simulink model "lti_id_0"  (R2018a)
settings: Solver=FixedStepAuto  StartTime=0.0  StopTime=5  FixedStep=0.0001  RelTol=1e-3
values from neighbouring files (symbols this model uses):
  b_eq = b_m + b_l/r^2    (= 1.5637748692e-05)    [PMSM_AyME.m]    (also in estabilidad_open_loop.m)
  J_eq = J_m + J_l/r^2    (= 5.65099476805e-06)    [PMSM_AyME.m]    (also in estabilidad_open_loop.m)
  L_q = 5.8E-3    (= 0.0058)    [PMSM_AyME.m]    (also in estabilidad_open_loop.m)
  lambda_m = 0.01546    [PMSM_AyME.m]    (also in estabilidad_open_loop.m)
  Pp = 3    [PMSM_AyME.m]    (also in estabilidad_open_loop.m)
  R_cq = -p_i*L_q    (= 29)    [PMSM_AyME.m]
  R_s = 1.02    [PMSM_AyME.m]    (also in estabilidad_open_loop.m)
settings Model: Creator=emiliano  LastModifiedBy=gino

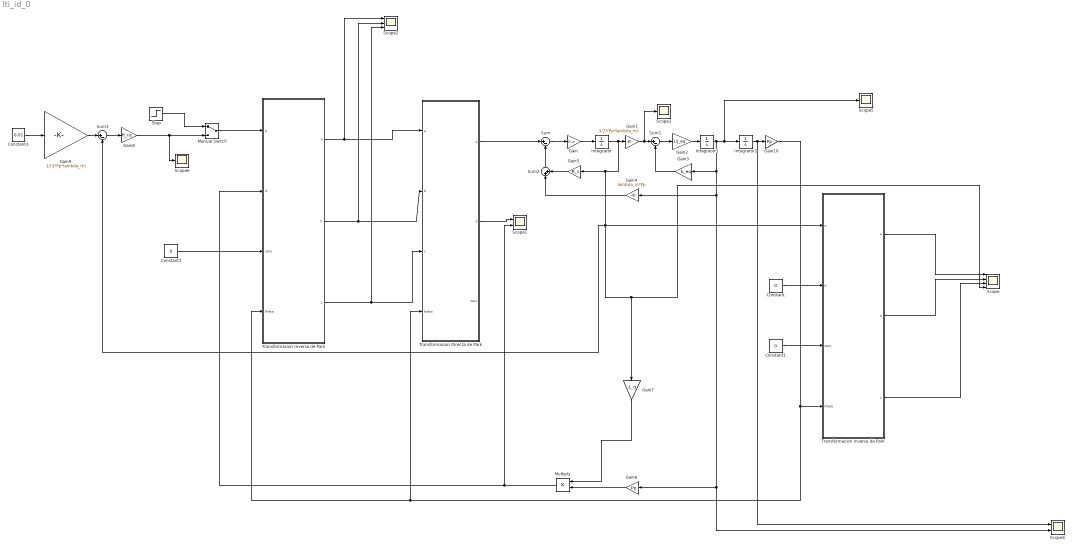
== system lti_id_0 ==
  Constant : Constant  Value=0
  Constant1 : Constant  Value=0
  Constant2 : Constant  Value=0
  Constant3 : Constant  Value=0.01
  Gain : Gain  Gain=1/L_q
  Gain1 : Gain  Gain=3/2*(Pp*lambda_m)
  Gain10 : Gain  Gain=Pp
  Gain2 : Gain  Gain=1/J_eq
  Gain3 : Gain  Gain=b_eq
  Gain4 : Gain  Gain=lambda_m*Pp
  Gain5 : Gain  Gain=R_s
  Gain6 : Gain  Gain=Pp
  Gain7 : Gain  Gain=-L_q
  Gain8 : Gain  Gain=R_cq
  Gain9 : Gain  Gain=2/(3*Pp*lambda_m)
  Integrator : Integrator
  Integrator1 : Integrator
  Integrator2 : Integrator
  Manual Switch : ManualSwitch
  Multiply : Product
  Scope : Scope  NumInputPorts=4
  Scope1 : Scope  NumInputPorts=2
  Scope2 : Scope  NumInputPorts=3
  Scope3 : Scope
  Scope4 : Scope  NumInputPorts=2
  Scope5 : Scope
  Scope6 : Scope
  Step : Step  After=20  SampleTime=0
  Sum : Sum  Inputs=|+-
  Sum1 : Sum  Inputs=|+-
  Sum2 : Sum  Inputs=|++
  Sum3 : Sum  Inputs=|+-
  Transformacion Directa de Park : MATLAB Function  TreatAsAtomicUnit=on
  Transformacion Inversa de Park : MATLAB Function  TreatAsAtomicUnit=on
  "Transformacion Inversa de Park " : MATLAB Function  TreatAsAtomicUnit=on
  wires:
  Sum/1 -> Gain/1
  Gain/1 -> Integrator/1
  Gain1/1 -> Scope3/1, Sum1/1
  Sum1/1 -> Gain2/1
  Gain2/1 -> Integrator1/1
  Integrator1/1 -> Scope4/2, Gain6/1, Gain4/1, Gain3/1, Scope5/1, Integrator2/1
  Gain3/1 -> Sum1/2
  Gain5/1 -> Sum2/2
  Sum2/1 -> Sum/2
  Gain4/1 -> Sum2/1
  Transformacion Directa de Park/1(q) -> Sum/1
  Integrator/1 -> Sum3/2, Scope/4, Gain7/1, Transformacion Inversa de Park/1(q), Gain5/1, Gain1/1
  Constant/1 -> Transformacion Inversa de Park/2(d)
  Constant1/1 -> Transformacion Inversa de Park/3(zero)
  Transformacion Inversa de Park/1(a) -> Scope/1
  Transformacion Inversa de Park/2(b) -> Scope/2
  Transformacion Inversa de Park/3(c) -> Scope/3
  Gain6/1 -> Multiply/2
  Gain7/1 -> Multiply/1
  Multiply/1 -> Scope1/2, "Transformacion Inversa de Park "/2(d)
  Constant2/1 -> "Transformacion Inversa de Park "/3(zero)
  Sum3/1 -> Gain8/1
  Constant3/1 -> Gain9/1
  Gain9/1 -> Sum3/1
  Transformacion Directa de Park/2(d) -> Scope1/1
  Gain10/1 -> Transformacion Directa de Park/4(theta), "Transformacion Inversa de Park "/4(theta), Transformacion Inversa de Park/4(theta)
  "Transformacion Inversa de Park "/1(a) -> Transformacion Directa de Park/1(a), Scope2/1
  "Transformacion Inversa de Park "/3(c) -> Transformacion Directa de Park/3(c), Scope2/3
  "Transformacion Inversa de Park "/2(b) -> Transformacion Directa de Park/2(b), Scope2/2
  Integrator2/1 -> Scope4/1, Gain10/1
  Manual Switch/1 -> "Transformacion Inversa de Park "/1(q)
  Gain8/1 -> Scope6/1, Manual Switch/2
  Step/1 -> Manual Switch/1

== matlab function lti_id_0/Transformacion Inversa de Park  ==
  data: q input; a output; d input; zero input; theta input; b output; c output
function [a, b, c] = inverse_park_transformation(q, d, zero, theta)
%Transformación inversa de Park
 
abc = [cos(theta)               sin(theta)              1
        cos(theta - 2*pi/3)     sin(theta - 2*pi/3)     1
        cos(theta + 2*pi/3)     sin(theta + 2*pi/3)     1] ...
    *   [q
        d
        zero];

a = abc(1);
b = abc(2);
c = abc(3);

end

== matlab function lti_id_0/Transformacion Directa de Park ==
  data: a input; q output; b input; c input; theta input; d output; zero output
function [q, d, zero] = park_transformation(a, b, c, theta)
%Transformación directa de Park
 
qdz = 2/3 * [cos(theta)     cos(theta - 2*pi/3)     cos(theta + 2*pi/3)
                    sin(theta)      sin(theta - 2*pi/3)     sin(theta + 2*pi/3)
                    1/2             1/2                     1/2] ...
                *   [a
                    b 
                    c];

q = qdz(1);
d = qdz(2);
zero = qdz(3);

end

== matlab function lti_id_0/Transformacion Inversa de Park ==
  data: q input; a output; d input; zero input; theta input; b output; c output
function [a, b, c] = inverse_park_transformation(q, d, zero, theta)
%Transformación inversa de Park
 
abc = [cos(theta)               sin(theta)              1
        cos(theta - 2*pi/3)     sin(theta - 2*pi/3)     1
        cos(theta + 2*pi/3)     sin(theta + 2*pi/3)     1] ...
    *   [q
        d
        zero];

a = abc(1);
b = abc(2);
c = abc(3);

end
